simulink model "model1c"  (R2014b)
settings: Solver=ode45  StartTime=0.0  StopTime=20.00  RelTol=1e-3
settings Model: Creator=Shane Reynolds  LastModifiedBy=Shane Reynolds

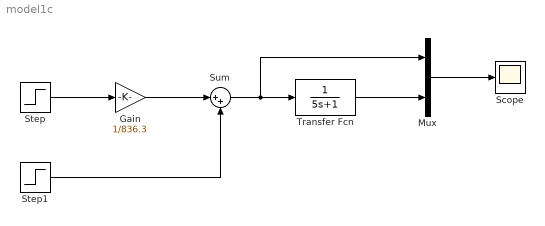
== system model1c ==
  Gain : Gain  Gain=1/836.3
  Mux : Mux  Inputs=2
  Scope : Scope
  Step : Step  After=2520  SampleTime=0
  Step1 : Step  After=10  SampleTime=0
  Sum : Sum  Inputs=|++
  Transfer Fcn : TransferFcn  Denominator=[5 1]
  wires:
  Step/1 -> Gain/1
  Gain/1 -> Sum/1
  Step1/1 -> Sum/2
  Sum/1 -> Mux/1, Transfer Fcn/1
  Mux/1 -> Scope/1
  Transfer Fcn/1 -> Mux/2
